simulink model "ARC_DTm"  (R2025b)
settings: Solver=FixedStepAuto  StartTime=0.0  StopTime=10080  FixedStep=1  RelTol=1e-3
PreLoadFcn:
  | %For Preload, set the working path
  | modelFolder = fileparts(which(bdroot));
  | addpath(genpath(modelFolder));
StartFcn:
  | tic
StopFcn:
  | fprintf("Sim Time: %.02f min", toc/60)
values from neighbouring files (symbols this model uses):
  batteryScenario = p.batteryScenario    [RUNSIM_ParameterSweep.m]    (also in _RUNSIM_ParameterSweep.m)
  Electricity_SalePriceModifier = 50/100    (= 0.5)    [RUNSIM_ParameterSweep.m]    (also in _RUNSIM_ParameterSweep.m)
  LUT = LUT_load.gamLUT    [RUNSIM_ParameterSweep.m]    (also in _RUNSIM_ParameterSweep.m)
  minimum_UF_system_flow = 5833    [RUNSIM_ParameterSweep.m]    (also in _RUNSIM_ParameterSweep.m)
  PROS1_recoveryrate = 61    [RUNSIM_ParameterSweep.m]    (also in _RUNSIM_ParameterSweep.m)
  PROS2_recoveryrate = 62    [RUNSIM_ParameterSweep.m]    (also in _RUNSIM_ParameterSweep.m)
  ROstabilization_time = p.ROstabilization_time    [RUNSIM_ParameterSweep.m]    (also in _RUNSIM_ParameterSweep.m)
  solarModifier = maximum_solar_generation / 300    [RUNSIM_ParameterSweep.m]    (also in _RUNSIM_ParameterSweep.m)
  TSRO_recoveryrate = 51    [RUNSIM_ParameterSweep.m]    (also in _RUNSIM_ParameterSweep.m)
  UF_RecoveryRate = 96    [RUNSIM_ParameterSweep.m]    (also in _RUNSIM_ParameterSweep.m)
undefined symbols (not defined in the file or in its folder): A_PROS1, A_PROS2, A_TSRO, B_PROS1, B_PROS2, B_TSRO, BW_Max_Time, BW_Max_Vol_gal, CEB_Max_Time, CEB_Max_Vol_gal, CIP_Max_Time, E, FF, h, L, w
libraries: simulink x40
(part 10 of 11)

== matlab function ARC_DTm/PROS2_4_Pump/MATLAB Function1 ==
  data: Q_des input; speed output; h_des input; power output
function [speed, power] = query_pump(Q_des, h_des)
% QUERY_PUMP Find pump speed, power, and efficiency given flow and head
%MUST UPDATE the pump_data call
%
% Inputs:
%   Q_des     - Desired flow rate (gpm)
%   h_des     - Desired added head (ft)
%   pump_data - Struct for a single pump (e.g. pump.pump_A)
%
% Outputs:
%   speed      - Interpolated speed
%   power      - Interpolated power
%   total_eff  - Interpolated total efficiency (%)
%   totalPower - Power demand accounting for efficiency (power / total_eff / 100)

persistent pump_data Q_min h_min speed_min  P_min
if isempty(pump_data)
    loaded = coder.load('Pumps\LookupTables.mat');
    pump_data = loaded.pump.RO_IS_pump;
    Q_min = min(pump_data.Q_grid(:));
    h_min = min(pump_data.H_grid(:));

    speed_min = interp2(pump_data.Q_grid, pump_data.H_grid, pump_data.speed_grid, Q_min, h_min, 'linear');
    P_min = interp2(pump_data.H_grid_pwr, pump_data.S_grid_pwr, pump_data.power_grid, h_min, speed_min, 'linear');

end

%zero flow conditions not present in the existing dataset.
if Q_des <= .1 * Q_min
    speed = 0;
    power = 0;
    total_eff = 0;
    return
end

% Normal lookup
speed = interp2(pump_data.Q_grid, pump_data.H_grid, ...
    pump_data.speed_grid, Q_des, h_des, 'linear');

if ~isnan(speed)
    power = interp2(pump_data.H_grid_pwr, pump_data.S_grid_pwr, ...
        pump_data.power_grid, h_des, speed, 'linear');
else
    power = NaN;
end

% Fallback only for low-end conditions
if isnan(speed) || isnan(power)
    if Q_des < Q_min       
        speed = speed_min / Q_min * Q_des;
         power = (speed / speed_min)^3 * P_min;

    else if h_des < h_min
        speed = speed_min * (h_des / h_min)^(1/2);
        power = (speed / speed_min)^3 * P_min;

    else
        speed = 0;
        power = 0;
    end


end


end

== matlab function ARC_DTm/PROS2_4/MATLAB Function1 ==
  data: W input; h input; dh output
function dh = hydDiameter(W,h)

dh = 2*h*W/(h+W);

== matlab function ARC_DTm/PROS2_4/MATLAB Function2 ==
  data: cperm input; cbrine output; Qperm input; Qbrine input; Qfeed input; cfeed input
function cbrine = fcn(cperm, Qperm, Qbrine, Qfeed, cfeed)

Wtot = Qfeed * cfeed;
Wperm = cperm * Qperm;

%account for NaN
if Qbrine > 0
cbrine = (Wtot - Wperm)/Qbrine;
else
    cbrine = 0;
end

== matlab function ARC_DTm/TSRO_Pump_1/MATLAB Function1 ==
  data: Q_des input; h_des input; power output
function power  = query_pump(Q_des, h_des)
% QUERY_PUMP Find pump speed, power, and efficiency given flow and head
%MUST UPDATE the pump_data call
%
% Inputs:
%   Q_des     - Desired flow rate (gpm)
%   h_des     - Desired added head (ft)
%   pump_data - Struct for a single pump (e.g. pump.pump_A)
%
% Outputs:
%   power      - Interpolated power
%   total_eff  - Interpolated total efficiency (%)
%   totalPower - Power demand accounting for efficiency (power / total_eff / 100)

persistent pump_data Q_min h_min P_min
if isempty(pump_data)
    loaded = coder.load('Pumps\LookupTables.mat');
    pump_data = loaded.pump.tsro;
    Q_min = min(pump_data.Q_grid(:));
    h_min = min(pump_data.H_grid(:));

    P_min = interp2(pump_data.Q_grid, pump_data.H_grid, pump_data.power_grid, h_min, Q_min, 'linear');

end

%zero flow conditions not present in the existing dataset.
if Q_des <= .1 * Q_min
    power = 0;
    return
end

% Normal lookup
power = interp2(pump_data.Q_grid, pump_data.H_grid, ...
    pump_data.power_grid, Q_des, h_des, 'linear');

if isnan(power)
    power = 0;
    return

end

== matlab function ARC_DTm/PROS2_4/Subsystem/MATLAB Function ==
  data: T input; Pfeed input; Pperm input; A input; B input; cfeed input; cperm_prev input; Jw_prev input; dh input; L input; u input; Jw output; cperm output; deltaPi_bar output
function [Jw, cperm, deltaPi_bar] = ROBehavior(T, Pfeed, Pperm, A, B, cfeed, cperm_prev,Jw_prev, dh, L, u)
   
    cmem = ConP(cfeed, T, dh, L, u, Jw_prev);
    [pi_feed] = osmPres(T,cmem);
    [pi_perm] = osmPres(T,cperm_prev);
    
    deltaPi_bar = pi_feed - pi_perm;
    [Jw, cperm] = solutionDiffusion(T, Pfeed, Pperm, A, B, cmem, cperm_prev, pi_feed, pi_perm);
end

== matlab function ARC_DTm/TSRO_1/MATLAB Function1 ==
  data: W input; h input; dh output
function dh = hydDiameter(W,h)

dh = 2*h*W/(h+W);

== matlab function ARC_DTm/TSRO_1/MATLAB Function2 ==
  data: cperm input; cbrine output; Qperm input; Qbrine input; Qfeed input; cfeed input
function cbrine = fcn(cperm, Qperm, Qbrine, Qfeed, cfeed)

Wtot = Qfeed * cfeed;
Wperm = cperm * Qperm;

%account for NaN
if Qbrine > 0
cbrine = (Wtot - Wperm)/Qbrine;
else
    cbrine = 0;
end

== matlab function ARC_DTm/TSRO_1/Subsystem/MATLAB Function ==
  data: T input; Pfeed input; Pperm input; A input; B input; cfeed input; cperm_prev input; Jw_prev input; dh input; L input; u input; Jw output; cperm output; deltaPi_bar output
function [Jw, cperm, deltaPi_bar] = ROBehavior(T, Pfeed, Pperm, A, B, cfeed, cperm_prev,Jw_prev, dh, L, u)
    
    
    cmem = ConP(cfeed, T, dh, L, u, Jw_prev);
    [pi_feed] = osmPres(T,cmem);
    [pi_perm] = osmPres(T,cperm_prev);
    deltaPi_bar = pi_feed - pi_perm;
    
    [Jw, cperm] = solutionDiffusion(T, Pfeed, Pperm, A, B, cmem, cperm_prev, pi_feed, pi_perm);
end

== matlab function ARC_DTm/TSRO_3/MATLAB Function1 ==
  data: W input; h input; dh output
function dh = hydDiameter(W,h)

dh = 2*h*W/(h+W);

== matlab function ARC_DTm/TSRO_3/MATLAB Function2 ==
  data: cperm input; cbrine output; Qperm input; Qbrine input; Qfeed input; cfeed input
function cbrine = fcn(cperm, Qperm, Qbrine, Qfeed, cfeed)

Wtot = Qfeed * cfeed;
Wperm = cperm * Qperm;

%account for NaN
if Qbrine > 0
cbrine = (Wtot - Wperm)/Qbrine;
else
    cbrine = 0;
end

== matlab function ARC_DTm/TSRO_3/Subsystem/MATLAB Function ==
  data: T input; Pfeed input; Pperm input; A input; B input; cfeed input; cperm_prev input; Jw_prev input; dh input; L input; u input; Jw output; cperm output; deltaPi_bar output
function [Jw, cperm, deltaPi_bar] = ROBehavior(T, Pfeed, Pperm, A, B, cfeed, cperm_prev,Jw_prev, dh, L, u)
    
    
    cmem = ConP(cfeed, T, dh, L, u, Jw_prev);

    [pi_feed] = osmPres(T,cmem);
    [pi_perm] = osmPres(T,cperm_prev);
    
    deltaPi_bar = pi_feed - pi_perm;
    [Jw, cperm] = solutionDiffusion(T, Pfeed, Pperm, A, B, cmem, cperm_prev, pi_feed, pi_perm);
end

== matlab function ARC_DTm/Product Water Tank/MATLAB Function ==
  settings: updateMethod=DISCRETE
  data: inflows input; newInflows output; outflows input; vol input; volStored input; upperVol input; lowerVol input; newOutflows output; dVdt output; t output; t input
function [newInflows, newOutflows, dVdt, t] = tankControllerLogic(inflows, outflows, vol, volStored, upperVol, lowerVol,t)
%determine tanks flows
inflowSum = sum(inflows); %total volume to be pushed into tank [FLOW]
outflowSum = sum(outflows); %total volume to be pulled from tank [FLOW]

%set timer to exist each time step
% persistent t
if isempty(t)
    t = 0;
end

if volStored >= upperVol
    t = 15;
elseif volStored <= lowerVol
    t = -15;
end


% disp("t = " + t)
%set flows to reach desired operating conditions
if t > 0 %reduce inflows
    newOutflows = outflows; %maintain outflows
    newInflows = zeros(length(inflows),1);
    inflowRatio = zeros(length(inflows),1); %preallocate variable
    newInflowSum = outflowSum * .95; %reduce Inflows to 95% outflows

    %maintain inflow ratios at new inflow level
    for i = 1:length(inflows)
        
        inflowRatio(i) = inflows(i)/inflowSum;
        newInflows(i) = newInflowSum * inflowRatio(i);
    end
    dVdt = newInflowSum - outflowSum;
    t = t-1; %reduce timer one step

elseif t < 0 %reduce outflows
    
    newInflows = inflows; %maintain inflows
  
    outflowRatio = zeros(length(outflows),1); %prellocate variable
    newOutflows = zeros(length(outflows),1);%preallocate variable
    newOutflowSum = inflowSum * .95; %reduce outflows to be below inflows

    %maintain inflow ratios at new inflow level
    for i = 1:length(outflows)
        outflowRatio(i) = outflows(i)/outflowSum;
        newOutflows(i) = newOutflowSum * outflowRatio(i);

    end
    dVdt = inflowSum - newOutflowSum;
    t = t+1; %reduce timer one step
    
else
    newInflows = inflows;
    newOutflows = outflows;
    dVdt = inflowSum - outflowSum;
end

%update stored volume

volStored = volStored + dVdt;

%if outside oeprating conditions, begin to adjust flows


end

== matlab function ARC_DTm/TSRO_2/MATLAB Function1 ==
  data: W input; h input; dh output
function dh = hydDiameter(W,h)

dh = 2*h*W/(h+W);

== matlab function ARC_DTm/TSRO_2/MATLAB Function2 ==
  data: cperm input; cbrine output; Qperm input; Qbrine input; Qfeed input; cfeed input
function cbrine = fcn(cperm, Qperm, Qbrine, Qfeed, cfeed)

Wtot = Qfeed * cfeed;
Wperm = cperm * Qperm;

%account for NaN
if Qbrine > 0
cbrine = (Wtot - Wperm)/Qbrine;
else
    cbrine = 0;
end

== matlab function ARC_DTm/TSRO_2/Subsystem/MATLAB Function ==
  data: T input; Pfeed input; Pperm input; A input; B input; cfeed input; cperm_prev input; Jw_prev input; dh input; L input; u input; Jw output; cperm output; deltaPi_bar output
function [Jw, cperm, deltaPi_bar] = ROBehavior(T, Pfeed, Pperm, A, B, cfeed, cperm_prev,Jw_prev, dh, L, u)
    
    
    cmem = ConP(cfeed, T, dh, L, u, Jw_prev);

    [pi_feed] = osmPres(T,cmem);
    [pi_perm] = osmPres(T,cperm_prev);
    
    deltaPi_bar = pi_feed - pi_perm;
    [Jw, cperm] = solutionDiffusion(T, Pfeed, Pperm, A, B, cmem, cperm_prev, pi_feed, pi_perm);
end

== matlab function ARC_DTm/TSRO_4/MATLAB Function1 ==
  data: W input; h input; dh output
function dh = hydDiameter(W,h)

dh = 2*h*W/(h+W);

== matlab function ARC_DTm/TSRO_4/MATLAB Function2 ==
  data: cperm input; cbrine output; Qperm input; Qbrine input; Qfeed input; cfeed input
function cbrine = fcn(cperm, Qperm, Qbrine, Qfeed, cfeed)

Wtot = Qfeed * cfeed;
Wperm = cperm * Qperm;

%account for NaN
if Qbrine > 0
cbrine = (Wtot - Wperm)/Qbrine;
else
    cbrine = 0;
end

== matlab function ARC_DTm/TSRO_4/Subsystem/MATLAB Function ==
  data: T input; Pfeed input; Pperm input; A input; B input; cfeed input; cperm_prev input; Jw_prev input; dh input; L input; u input; Jw output; cperm output; deltaPi_bar output
function [Jw, cperm, deltaPi_bar] = ROBehavior(T, Pfeed, Pperm, A, B, cfeed, cperm_prev,Jw_prev, dh, L, u)
    
    
    cmem = ConP(cfeed, T, dh, L, u, Jw_prev);

    [pi_feed] = osmPres(T,cmem);
    [pi_perm] = osmPres(T,cperm_prev);
    
    deltaPi_bar = pi_feed - pi_perm;
    [Jw, cperm] = solutionDiffusion(T, Pfeed, Pperm, A, B, cmem, cperm_prev, pi_feed, pi_perm);
end

== matlab function ARC_DTm/TSRO_Pump_3/MATLAB Function1 ==
  data: Q_des input; h_des input; power output
function power  = query_pump(Q_des, h_des)
% QUERY_PUMP Find pump speed, power, and efficiency given flow and head
%MUST UPDATE the pump_data call
%
% Inputs:
%   Q_des     - Desired flow rate (gpm)
%   h_des     - Desired added head (ft)
%   pump_data - Struct for a single pump (e.g. pump.pump_A)
%
% Outputs:
%   power      - Interpolated power
%   total_eff  - Interpolated total efficiency (%)
%   totalPower - Power demand accounting for efficiency (power / total_eff / 100)

persistent pump_data Q_min h_min P_min
if isempty(pump_data)
    loaded = coder.load('Pumps\LookupTables.mat');
    pump_data = loaded.pump.tsro;
    Q_min = min(pump_data.Q_grid(:));
    h_min = min(pump_data.H_grid(:));

    P_min = interp2(pump_data.Q_grid, pump_data.H_grid, pump_data.power_grid, h_min, Q_min, 'linear');

end

%zero flow conditions not present in the existing dataset.
if Q_des <= .1 * Q_min
    power = 0;
    return
end

% Normal lookup
power = interp2(pump_data.Q_grid, pump_data.H_grid, ...
    pump_data.power_grid, Q_des, h_des, 'linear');

if isnan(power)
    power = 0;
    return

end

== matlab function ARC_DTm/TSRO_Pump_4/MATLAB Function1 ==
  data: Q_des input; h_des input; power output
function power  = query_pump(Q_des, h_des)
% QUERY_PUMP Find pump speed, power, and efficiency given flow and head
%MUST UPDATE the pump_data call
%
% Inputs:
%   Q_des     - Desired flow rate (gpm)
%   h_des     - Desired added head (ft)
%   pump_data - Struct for a single pump (e.g. pump.pump_A)
%
% Outputs:
%   power      - Interpolated power
%   total_eff  - Interpolated total efficiency (%)
%   totalPower - Power demand accounting for efficiency (power / total_eff / 100)

persistent pump_data Q_min h_min P_min
if isempty(pump_data)
    loaded = coder.load('Pumps\LookupTables.mat');
    pump_data = loaded.pump.tsro;
    Q_min = min(pump_data.Q_grid(:));
    h_min = min(pump_data.H_grid(:));

    P_min = interp2(pump_data.Q_grid, pump_data.H_grid, pump_data.power_grid, h_min, Q_min, 'linear');

end

%zero flow conditions not present in the existing dataset.
if Q_des <= .1 * Q_min
    power = 0;
    return
end

% Normal lookup
power = interp2(pump_data.Q_grid, pump_data.H_grid, ...
    pump_data.power_grid, Q_des, h_des, 'linear');

if isnan(power)
    power = 0;
    return

end

== stateflow chart ARC_DTm/UF Maintenance Coordinator/Sample_Stateflows ==
  settings: sampleTime=1  executeAtInitialization=1
  note: Unit State Machine — FIFO Maintenance Dispatch
      | This chart controls a single filtration unit through four operational states: Standby, Running, Await_Maintenance, BW_Maintenance, and CEB_Maintenance.
      | The unit begins in Standby, awaiting a startup command from the central dispatcher. Once commanded on, it enters Running, where it operates normally and tracks cumulative downtime. If a maintenance request is triggered, the unit transitions to Await_Maintenance, remaining online until the dispatcher confirms it can be released.
      | Two maintenance sequences are supported. A Backwash (BW) is a fixed-duration event (4 timesteps). A Chemically Enhanced Backwash (CEB) is a stochastic event lasting between 30 and 90 timesteps, sampled from a uniform distribution at entry. CEB is always followed by a BW cycle.
      | Upon completion of maintenance, the unit returns to Standby and re-enters the startup queue at the back, consistent with FIFO dispatching logic.
  note: Unit_cmd = 1 for running, 0 for off.
  state Standby
    during:
    %Unit is off, but awaiting startup.
    unit_in_startup_queue = 1;
    unit_in_operation = 0;
    %Ensure that the maintenance resets are occuring.
    maintenance_completion_indicator = 0;
  state Running
    entry:
    %Reset downtime timer
    cycle_downtime = 0;
    during:
    %Unit on, not in maint queue.
    unit_in_operation = 1;
    unit_in_maint_queue = 0;
  state Await_standby
    %Unit , Enter maint Queue
    during:
    unit_in_operation = 0;
    unit_in_maint_queue = 1;
  state Await_maintenance
    %Unit stays on, Enter maint Queue
    during:
    unit_in_operation = 1;
    unit_in_maint_queue = 1;
  state CEB_Maintenance
    %Unit is in chemically enhanced backwash. After CEB, do BW.
    %At start, determine a maintenance time within a uniform range of 30-60 min.
    entry:
    needed_maint_time = 30 + (60-30) * rand();
    %Exit state when time in maintenance is >= expected time.
    during:
    unit_in_operation = -1; %unit in maintenance
    %update maintenance time every step.
    cycle_downtime = cycle_downtime + 1;
  state BW_Maintenance
    entry:
    needed_maint_time = 1.5;
    %Exit state when time in maintenance is >= expected time.
    during:
    unit_in_operation = -1; %unit in maintenance
    %update maintenance time every step.
    cycle_downtime = cycle_downtime + 1;
    %ensure that the CEB is not continually reseting.
    maintenance_completion_indicator = 0;
  note: Maintenance Completion Indicator represents a signal to reset the counters at the UF unit tracking backwash cycles (signal = 2) and time in operations (signal = 1). These are pulse signals that reset integrators.
  (default) -> Running
  Standby -> Running : [startup_cmd == 1]{unit_in_startup_queue = 0;}
  Running -> (junction 44) [order 2] : [standby_cmd == 1]
  Running -> Await_maintenance [order 1] : [maint_req ~=0]
  (junction 22) -> Standby
  Await_standby -> (junction 47) : [standby_cmd == 1 && maint_cmd == 1]
  (junction 47) -> (junction 11)
  (junction 44) -> Await_standby
  Await_maintenance -> (junction 11) [order 2] : [maint_req == 1 && maint_cmd == 1] {unit_in_maint_queue = 0;}
  (junction 11) -> BW_Maintenance
  Await_maintenance -> CEB_Maintenance [order 1] : [maint_req == 2 && maint_cmd ==1]
  CEB_Maintenance -> BW_Maintenance : [after(needed_maint_time, tick)]{maintenance_completion_indicator = 2;}
  BW_Maintenance -> (junction 22) : [after(needed_maint_time, tick)]
      | {maintenance_completion_indicator = 1;}
  data: maint_cmd input; maint_req input; standby_cmd input; startup_cmd input; unit_in_maint_queue output; unit_in_startup_queue output; cycle_downtime local; needed_maint_time local; unit_in_operation output; maintenance_completion_indicator output

== matlab function ARC_DTm/UF_Feed_Manifold/UF_Dispatcher ==
  data: flows output; max_flow_per_unit input; flow_actual input; Number_in_service output; flow_setpoint input; prev_flows input; demanded_flows output
function [flows, Number_in_service, demanded_flows] = UF_Dispatcher(max_flow_per_unit, flow_actual, flow_setpoint, prev_flows)

num_units_available = 10; 
flows = zeros( num_units_available,1);
demanded_flows = zeros(num_units_available,1);

current_units = sum(prev_flows>0);
target_units = min(ceil(flow_setpoint / max_flow_per_unit), num_units_available);
% Unit count driven by setpoint

    %during rampdown, avoid shutting off all units immediately
    if flow_setpoint == 0 && flow_actual ~= 0
        Number_in_service = max(target_units, current_units);
    else
        Number_in_service = target_units;
    end

% Target each unit is heading toward (based on setpoint)
demanded_flows(1:Number_in_service) = flow_setpoint / Number_in_service;

% Change in total actual flow this timestep (this should be throttled by
% rate limiter) on flow_actual.
delta_Q_total = flow_actual - sum(prev_flows); %total change in flow this timestep
avg_delta_Q_unit = delta_Q_total/Number_in_service; %benchmark to limit rate change.

% Distribute that delta evenly across active units, move toward demanded
delta_Q_unit_demanded = zeros(num_units_available,1); %demanded change in flows to reach setpoint
delta_Q = zeros(num_units_available,1); %actual change in flows this step.
for i = 1:num_units_available

        %get demanded change in flows.
        delta_Q_unit_demanded(i) = demanded_flows(i) - prev_flows(i);  
         
        delta_Q(i) = sign(delta_Q_unit_demanded(i)) * min(abs(delta_Q_unit_demanded(i)), abs(delta_Q_total/Number_in_service));


        flows(i) = prev_flows(i) + delta_Q(i);
        

        delta_Q_total = delta_Q_total - delta_Q(i);
end

end

== matlab function ARC_DTm/Product Water Tank/Tank Storage/Manage Overflows/Reduce to Zero ==
  data: u input; y output
function y = fcn(u)
    if u > 0 
        y = u -1;
        
    elseif u < 0
        y = u+1;
    else
        y = 0;
    end
    fprintf("Timer = ", +y)
end

== matlab function ARC_DTm/UF Maintenance Coordinator/UF_FIFO_Coordinator ==
  data: startup_req input size=[10 1]; maint_req input size=[10 1]; operating_states input; startup_cmd output size=[10 1]; flows input; maint_cmd output size=[10 1]; shutdown_cmd output size=[10 1]; assigned_flows output
function [startup_cmd, maint_cmd, shutdown_cmd,  assigned_flows] = ...
        FIFO_coordinator(startup_req, maint_req, operating_states, flows)
% ========================================
%  FIFO_coordinator  —  Startup / Maintenance / Shutdown coordinator
%
%  Manages 10 units so that exactly `demanded_units` are running at all
%  times. All queues are strict FIFO. Designed for use as a MATLAB
%  Function block inside Simulink (fixed-step discrete, Ts = 1).
%
%  INPUTS
%  startup_req   [10×1]  bool   unit is in Standby, requesting startup
%  maint_req   [10×1]  int    0=none, 1=BW request, 2=CEB request
%  unit_in_operation  [10×1]  int    -1=in active maint, 0=standby, 1=running/await_maint
%  demanded_units   scalar  int    how many units should be online right now
%
%  OUTPUTS
%  startup_cmd    [10×1]  bool  tell unit to leave Standby to Running
%  maint_cmd  [10×1]  bool  tell unit to leave Await_Maintenance to BW/CEB
%  shutdown_cmd  [10×1]  bool tell unit to leave Running to Standby
%  running_count  scalar int   number of units currently online (operation == 1)
%
%  UNIT STATE ENCODING (unit_in_operation)
%   1:  Running OR Await_Maintenance  (online, contributing to flow)
%   0:  Standby                       (offline, may be in startup queue)
%  -1:  BW_Maintenance or CEB_Maint  (offline, maintenance in progress)
%
%  COORDINATOR DECISION ORDER (each timestep):
%   1. Enqueue   — register new startup/maint requests into FIFO queues
%   2. Shed Load — if running_count > demanded, release maint or shutdown
%   3. Maint     — if slot open and safe, release front of maint queue
%   4. Startup   — if running_count < demanded, pop from startup queue
% ==================================

N = 10;
demanded_units = sum(flows>0); %from flow logic, determine number of units needed
% ── Persistent state (survives across Simulink timesteps) ─────────────────
persistent startup_queue;   % ordered list of unit indices awaiting startup
persistent maint_queue;     % ordered list of unit indices awaiting maintenance

if isempty(startup_queue)
    startup_queue = [];
    maint_queue   = [];
end



% ── Initialise output vectors ─────────────────────────────────────────────
startup_cmd  = zeros(N, 1);
maint_cmd = zeros(N, 1);
shutdown_cmd = zeros(N, 1);

% ── Derived counts from unit feedback signals ─────────────────────────────
running_count = sum(operating_states == 1);   % online units
active_maint_count = sum(operating_states == -1);  % unit in BW or CEB
% =======================
% STEP 1 — Add to queues
%   Add newly requesting units to the back of their respective queues.
%   Guards prevent double-enqueuing.
% ================================
for i = 1:N

    % Startup queue: unit must be in Standby (op==0) and not already queued
    if startup_req(i) && ~ismember(i, startup_queue) && operating_states(i) == 0
        startup_queue(end+1) = i;
    end

    % Maint queue: unit must be online (operating state ==1) and not already queued
    if maint_req(i) ~= 0 && ~ismember(i, maint_queue) && operating_states(i) == 1
        maint_queue(end+1) = i; 
    end

end

% =========================================================================
% STEP 2 — SHED LOAD
%   If too many units are online, bring count down to demanded_units.
%
%   Priority 1: units already in Await_Maintenance (maint_queue front)
%               , then issue maint_cmd immediately; they go offline with 0 flow.
%               Only possible if no other unit is currently in active maint
%               (one-at-a-time constraint).
%               After issuing maint_cmd, continue immediately to re-evaluate
%               the while condition — do NOT fall into shutdown branch.
%
%   Priority 2: pure Running units → issue shutdown_cmd (lowest index first
%               among units not in maint_queue, to preserve FIFO integrity).
%               already_shutdown tracks victims within this timestep since
%               unit_in_operation won't update until next step.
% =========================================================================
already_shutdown = zeros(N, 1);   % prevents double-shutdown in same timestep
already_maint    = zeros(N, 1);   % tracks units sent to maint this timestep
                                  % (unit_in_operation won't update until next
                                  %  step, so we must exclude them manually)

%Case 1. turn down requires shut down of units                                  
while running_count > demanded_units

    % Priority 1: shed via maint queue if slot is open
    if ~isempty(maint_queue) && active_maint_count == 0
        victim                = maint_queue(1);
        maint_queue(1)        = [];
        maint_cmd(victim)     = 1;
        already_maint(victim) = 1;   % exclude from shutdown candidates
        running_count         = running_count - 1;
        active_maint_count    = active_maint_count + 1;
        continue;   % re-evaluate while condition; skip shutdown branch
    end

    % Priority 2: shutdown lowest-index running unit not in maint queue
    %   Exclude units already sent to maint this step (still show op==1)
    candidates = find(operating_states == 1         & ...
                      ~ismember((1:N)', maint_queue) & ...
                      ~already_shutdown  & ...
                      ~already_maint);
    if ~isempty(candidates)
        victim   = candidates(1);
        shutdown_cmd(victim) = 1;
        already_shutdown(victim)= 1;
        startup_queue(startup_queue == victim) = [];
        running_count = running_count - 1;
    else
        break;   % nothing left to shed this step
    end

end

% =======================================================
% STEP 3 — RELEASE MAINTENANCE
%   Conditions to release the front of the maint queue:
%     a) at least one unit is in the maint queue
%     b) no unit is currently in active maintenance (one-at-a-time)
%     c) there is a replacement unit on standby
% =========================================================
if ~isempty(maint_queue) && ...
   ~isempty(startup_queue) &&...
   active_maint_count == 0  

    next_maint_unit = maint_queue(1);
    maint_queue(1) = [];
    maint_cmd(next_maint_unit)  = 1;

    next_startup_unit = startup_queue(1);
    startup_queue(1) = [];
    startup_cmd(next_startup_unit) = 1;
    active_maint_count = active_maint_count + 1;

    % active_maint_count would increment next step via unit feedback
    % also, running_count remains unchanged as a new unit comes online.

end



% ============================================
% STEP 4 — START UNITS
%   If running_count is below demand, pop from the front of the startup
%   queue and issue startup_cmd. Repeat until balanced or queue exhausted.
% =========================================================
while running_count < demanded_units && ~isempty(startup_queue)

    next_startup_unit = startup_queue(1);
    startup_queue(1)        = [];
    startup_cmd(next_startup_unit)  = 1;
    running_count           = running_count + 1;
    % unit_in_operation will rise to 1 next step via unit Stateflow

end

% =========================================================================
% STEP 5 - Assign Flows
% Based on flows vector, distribute the flows per unit to the units that
% are on. 
%===============================================================
assigned_flows = zeros(N,1); %initialize object

online_units = find(operating_states==1); %array of indices for online units

if isempty(online_units)
    assigned_flows = zeros(N,1);
else

flows_available = flows(flows>0); %flows by unit by dispatcher

number_to_assign = min(length(online_units), length(flows_available)); %only assign the minimum

for i = 1:number_to_assign
    assigned_flows(online_units(i)) = flows_available(i);
end

end

end % function

== matlab function ARC_DTm/PRO Concentrate Manifold/Number TSRO Units ==
  data: flows output; max_flow_per_unit input; flow_actual input; Number_in_service output; flow_setpoint input; prev_flows input; Stabilization_Time input; ROstabilization_time input
function [flows, Number_in_service] = TSROUnits(max_flow_per_unit, flow_actual, flow_setpoint, prev_flows, Stabilization_Time,ROstabilization_time)

flows = zeros( 4,1);
demanded_flows = zeros(4,1);

current_units = sum(prev_flows>0);
target_units = min(ceil(flow_setpoint / max_flow_per_unit), 4);
% Unit count driven by setpoint
if Stabilization_Time >= ROstabilization_time

    %during rampdown, avoid shutting off all units immediately
    if flow_setpoint == 0 && flow_actual ~= 0
        Number_in_service = max(target_units, current_units);
    else
        Number_in_service = target_units;
    end
else
    Number_in_service = 2;
end

% Target each unit is heading toward (based on setpoint)
demanded_flows(1:Number_in_service) = flow_setpoint / Number_in_service;

% Change in total actual flow this timestep (this should be throttled by
% rate limiter) on flow_actual.
delta_Q_total = flow_actual - sum(prev_flows); %total change in flow this timestep
avg_delta_Q_unit = delta_Q_total/Number_in_service; %benchmark to limit rate change.

% Distribute that delta evenly across active units, move toward demanded
delta_Q_unit_demanded = zeros(4,1); %demanded change in flows to reach setpoint
delta_Q = zeros(4,1); %actual change in flows this step.
for i = 1:4

        %get demanded change in flows.
        delta_Q_unit_demanded(i) = demanded_flows(i) - prev_flows(i);  
         
        delta_Q(i) = sign(delta_Q_unit_demanded(i)) * min(abs(delta_Q_unit_demanded(i)), abs(delta_Q_total/Number_in_service));


        flows(i) = prev_flows(i) + delta_Q(i);
        

        delta_Q_total = delta_Q_total - delta_Q(i);
end

end

== matlab function ARC_DTm/UF Maintenance Coordinator/UF_State_Tracker ==
  data: in_startup_queue output; in_maint_queue output; startup_cmd input; operations_states output; maint_cmd input; shutdown_cmd input; maint_req input; maintenance_completion_indicators output
function [ in_startup_queue, in_maint_queue,operations_states, maintenance_completion_indicators] = ...
          UF_Operating_States(startup_cmd, maint_cmd, shutdown_cmd, maint_req)
% UF Maintenance Tracker
%This function is a more efficient way to operate N identical stateflow
%diagrams representing UF maintenance cycles. 

%Note that the ordering of the queue is handled within the Coordinator
%function, and the persistence of queueing order is also contained there.
% -------------------------------------------------------------------------

% ___ Inputs - From Coordinator___
%   startup_cmd  [10x1] logical, move units in queue Standby to Running
%   maint_cmd [10x1] logical, move units in queue Await_Maint to Maintenance
%   shutdown_cmd [10x1] logical, move units in queue Running/Await_Maint to Standby

% ___Inputs - from units___
% maintenance_requests [10x1] state-based triggers. move units from Running
% to Await_Maint
%   [0 (no maint request), 1 (Backwash request), 2 (Chemically-Enahnced BW
%   Req)]

% ___OUTPUTS - to coordinator___
%   operation_states [10x1] int: -1=active maint, 0=standby, 1=online
%   startup_queue  [10x1] logical
%   maint_queue [10x1] logical

%___Outputs - to units___
%   maintenance_completion_indicators  [10x1] int: 0=none, 1=BW complete, 2=CEB complete

% ___Internal Vectors___
%   needed_maint_time [10x1] double, stochastic constants for the duration
%   of a maintenance activity.
%   time_in_maintenance_p [10x1] double, maintenance duration

% -------------------------------------------------------------------------

N = 10;

% operations state constants. Use doubles for MATLAB Function block compatibility.
STANDBY = 0;
RUNNING = 1;
AWAIT_MAINTENANCE = 2;
BW_MAINTENANCE = -1;
CEB_MAINTENANCE = -2;



%Define and initialize persistent variables
%Note, in simulink, persistent variables cannot be used as function outputs, only internal state variables
persistent operations_states_p;
persistent time_in_maintenance_p;
persistent needed_maint_time_p;


if isempty(operations_states_p)

    % all units start in Standby
    operations_states_p = zeros(N,1); 
    time_in_maintenance_p = zeros(N,1); 
    needed_maint_time_p = zeros(N,1);
    


end

% Initialize outputs each tick. Note that the queues are stored in the
% UFCoordinator Function
maintenance_completion_indicators = zeros(N,1);
in_maint_queue = zeros(N,1);
in_startup_queue = zeros(N,1); 

%for each unit
for i = 1:N
    
    %determine the operating state
    switch operations_states_p(i)

        case STANDBY %state == 0

            % Stateflow Standby/during equivalent:
            %   unit is off, awaiting startup.
            
            %while unit is in standby:

            operations_states_p(i) = STANDBY; %not operating
            in_startup_queue(i) = 1; %in startup queue
            in_maint_queue(i) = 0; %no maintenance request

            if startup_cmd(i)
                operations_states_p(i) = RUNNING;
                in_startup_queue(i) = 0;
            end

        case RUNNING %state == 1
            % Stateflow Running/entry and during equivalent:
            % unit online, not in maintenance queue.

            operations_states_p(i) = RUNNING; %in operation

            %not in any queue
            in_startup_queue(i) = 0;
            in_maint_queue(i) = 0;
            
            %when shutdown command (during rampdown) issued by coordinator
            if shutdown_cmd(i)

                operations_states_p(i) = STANDBY; %no longer operating
                in_startup_queue(i) = 1; %enter startup queue

            %If  unit hits maintenance threshold(s)
            elseif maint_req(i) ~= 0

                %send out maintenance request. 
                operations_states_p(i) = AWAIT_MAINTENANCE;
                in_maint_queue(i) = 1;
            end

        case AWAIT_MAINTENANCE
            % Unit remains online while waiting for coordinator permission.
            operations_states_p(i) = AWAIT_MAINTENANCE;

            %Only in maintenance queue
            in_startup_queue(i) = 0;
            in_maint_queue(i) = 1;

            % If the shutdown command is issued (such as during rampdown)
            if shutdown_cmd(i)
                
                %enter standby and remove self from maintenance queue
                operations_states_p(i) = STANDBY;
                operations_states_p(i) = 0;
                in_startup_queue(i) = 1;
                in_maint_queue(i) = 0;
            
            %Otherwise, if the command to enter maintenance is issued:
            elseif maint_cmd(i)
                in_maint_queue(i) = 0; %remove self from maintenance queue
                time_in_maintenance_p(i) = 0; %initialize time in maintenance tracker
                
                %if unit requested CEB maintenance
                if maint_req(i) == 2
                    operations_states_p(i) = CEB_MAINTENANCE; 
                    % Stateflow entry action:
                    %   needed_maint_time = 30 + (60-30)*rand();
                    needed_maint_time_p(i) = 30 + 30*rand(); %set time to 30-60 mins

                    %Otherwise, if BW is requested (more common)
                else
                    operations_states_p(i) = BW_MAINTENANCE;
                    % Stateflow entry action:
                    %   needed_maint_time = 1.5;
                    needed_maint_time_p(i) = 1.5;  %set time to ~2 min. 
                end
            end

        case CEB_MAINTENANCE
            % Active CEB: unit offline, downtime accumulates.
            operations_states_p(i) = CEB_MAINTENANCE;
            in_startup_queue(i) = 0;
            in_maint_queue(i) = 0;
            time_in_maintenance_p(i) = time_in_maintenance_p(i) + 1;

            if time_in_maintenance_p(i) >= needed_maint_time_p(i)
                % CEB complete; original chart indicates CEB is followed by BW.
                maintenance_completion_indicators(i) = 2;
                operations_states_p(i) = BW_MAINTENANCE;

                time_in_maintenance_p(i) = 0;
                needed_maint_time_p(i) = 1.5;
            end

        case BW_MAINTENANCE
            % Active BW: unit offline, downtime accumulates.
            operations_states_p(i) = BW_MAINTENANCE;
            in_startup_queue(i) = 0;
            in_maint_queue(i) = 0;
            time_in_maintenance_p(i) = time_in_maintenance_p(i) + 1;

            if time_in_maintenance_p(i) >= needed_maint_time_p(i)
                % BW complete; return to Standby/startup queue.
                maintenance_completion_indicators(i) = 1;
                operations_states_p(i) = STANDBY;
                time_in_maintenance_p(i) = 0;
                needed_maint_time_p(i) = 0;
            end

        otherwise
            % Defensive recovery for invalid state values.
            operations_states_p(i) = STANDBY;
            time_in_maintenance_p(i) = 0;
            needed_maint_time_p(i) = 0;
            operations_states_p(i) = 0;
            in_startup_queue(i) = 1;
            in_maint_queue(i) = 0;
    end
end

% Refresh diagnostic outputs after state updates.
operations_states = sign(operations_states_p);


end

== matlab function ARC_DTm/UF Maintenance Coordinator/arhive/MATLAB Function ==
  data: startup_req input size=[10 1]; maint_req input size=[10 1]; unit_in_operation input; startup_cmd output size=[10 1]; demanded_units input; maint_cmd output size=[10 1]; shutdown_cmd output size=[10 1]; running_count output
function [startup_cmd, maint_cmd, shutdown_cmd, running_count] = ...
        FIFO_coordinator(startup_req, maint_req, unit_in_operation, demanded_units)
% =========================================================================
%  FIFO_coordinator  —  Startup / Maintenance / Shutdown coordinator
%
%  Manages 10 units so that exactly `demanded_units` are running at all
%  times. All queues are strict FIFO. Designed for use as a MATLAB
%  Function block inside Simulink (fixed-step discrete, Ts = 1).
%
%  INPUTS
%  startup_req        [10×1]  bool   unit is in Standby, requesting startup
%  maint_req          [10×1]  int    0=none, 1=BW request, 2=CEB request
%  unit_in_operation  [10×1]  int    -1=in active maint, 0=standby, 1=running/await_maint
%  demanded_units     scalar  int    how many units should be online right now
%
%  OUTPUTS
%  startup_cmd        [10×1]  bool   tell unit to leave Standby → Running
%  maint_cmd          [10×1]  bool   tell unit to leave Await_Maintenance → BW/CEB
%  shutdown_cmd       [10×1]  bool   tell unit to leave Running → Standby
%  running_count      scalar  int    number of units currently online (operation == 1)
%
%  UNIT STATE ENCODING (unit_in_operation)
%   1:  Running OR Await_Maintenance  (online, contributing to flow)
%   0:  Standby                       (offline, may be in startup queue)
%  -1:  BW_Maintenance or CEB_Maint  (offline, maintenance in progress)
%
%  COORDINATOR DECISION ORDER (each timestep):
%   1. Enqueue   — register new startup/maint requests into FIFO queues
%   2. Shed Load — if running_count > demanded, release maint or shutdown
%   3. Maint     — if slot open and safe, release front of maint queue
%   4. Startup   — if running_count < demanded, pop from startup queue
% =========================================================================

N = 10;
% ── Persistent state (survives across Simulink timesteps) ─────────────────
persistent startup_queue;   % ordered list of unit indices awaiting startup
persistent maint_queue;     % ordered list of unit indices awaiting maintenance

if isempty(startup_queue)
    startup_queue = [];
    maint_queue   = [];
end



% ── Initialise output vectors ─────────────────────────────────────────────
startup_cmd  = false(N, 1);
maint_cmd    = false(N, 1);
shutdown_cmd = false(N, 1);

% ── Derived counts from unit feedback signals ─────────────────────────────
running_count      = sum(unit_in_operation == 1);   % online units
active_maint_count = sum(unit_in_operation == -1);  % units in BW or CEB

% =========================================================================
% STEP 1 — ENQUEUE
%   Add newly requesting units to the back of their respective queues.
%   Guards prevent double-enqueuing.
% =========================================================================
for i = 1:N

    % Startup queue: unit must be in Standby (op==0) and not already queued
    if startup_req(i) && ~ismember(i, startup_queue) && unit_in_operation(i) == 0
        startup_queue(end+1) = i; %#ok<AGROW>
    end

    % Maint queue: unit must be online (op==1) and not already queued
    if maint_req(i) ~= 0 && ~ismember(i, maint_queue) && unit_in_operation(i) == 1
        maint_queue(end+1) = i; %#ok<AGROW>
    end

end

% =========================================================================
% STEP 2 — SHED LOAD
%   If too many units are online, bring count down to demanded_units.
%
%   Priority 1: units already in Await_Maintenance (maint_queue front)
%               → issue maint_cmd immediately; they go offline with 0 flow.
%               Only possible if no other unit is currently in active maint
%               (one-at-a-time constraint).
%               After issuing maint_cmd, continue immediately to re-evaluate
%               the while condition — do NOT fall into shutdown branch.
%
%   Priority 2: pure Running units → issue shutdown_cmd (lowest index first
%               among units not in maint_queue, to preserve FIFO integrity).
%               already_shutdown tracks victims within this timestep since
%               unit_in_operation won't update until next step.
% =========================================================================
already_shutdown = false(N, 1);   % prevents double-shutdown in same timestep
already_maint    = false(N, 1);   % tracks units sent to maint this timestep
                                  % (unit_in_operation won't update until next
                                  %  step, so we must exclude them manually)

while running_count > demanded_units

    % Priority 1: shed via maint queue if slot is open
    if ~isempty(maint_queue) && active_maint_count == 0
        victim                = maint_queue(1);
        maint_queue(1)        = [];
        maint_cmd(victim)     = true;
        already_maint(victim) = true;   % exclude from shutdown candidates
        running_count         = running_count - 1;
        active_maint_count    = active_maint_count + 1;
        continue;   % re-evaluate while condition; skip shutdown branch
    end

    % Priority 2: shutdown lowest-index running unit not in maint queue
    %   Exclude units already sent to maint this step (still show op==1)
    candidates = find(unit_in_operation == 1         & ...
                      ~ismember((1:N)', maint_queue) & ...
                      ~already_shutdown              & ...
                      ~already_maint);
    if ~isempty(candidates)
        victim                   = candidates(1);
        shutdown_cmd(victim)     = true;
        already_shutdown(victim) = true;
        startup_queue(startup_queue == victim) = [];
        running_count            = running_count - 1;
    else
        break;   % nothing left to shed this step
    end

end

% =========================================================================
% STEP 3 — RELEASE MAINTENANCE
%   Conditions to release the front of the maint queue:
%     a) at least one unit is in the maint queue
%     b) no unit is currently in active maintenance (one-at-a-time)
%     c) releasing won't drop running_count below demanded_units
%        (the unit goes offline during maint)
% =========================================================================
if ~isempty(maint_queue)         && ...
   active_maint_count == 0       && ...
   (running_count - 1) >= demanded_units

    next_unit = maint_queue(1);
    maint_queue(1)        = [];
    maint_cmd(next_unit)  = true;
    running_count         = running_count - 1;
    % active_maint_count would increment next step via unit feedback

end

% =========================================================================
% STEP 4 — START UNITS
%   If running_count is below demand, pop from the front of the startup
%   queue and issue startup_cmd. Repeat until balanced or queue exhausted.
% =========================================================================
while running_count < demanded_units && ~isempty(startup_queue)

    next_unit = startup_queue(1);
    startup_queue(1)        = [];
    startup_cmd(next_unit)  = true;
    running_count           = running_count + 1;
    % unit_in_operation will rise to 1 next step via unit Stateflow

end

end % function

== stateflow chart ARC_DTm/UF Maintenance Coordinator/arhive/UF_Operation State_1/UF1_Maintenance State ==
  settings: sampleTime=1  executeAtInitialization=1
  note: Unit State Machine — FIFO Maintenance Dispatch
      | This chart controls a single filtration unit through four operational states: Standby, Running, Await_Maintenance, BW_Maintenance, and CEB_Maintenance.
      | The unit begins in Standby, awaiting a startup command from the central dispatcher. Once commanded on, it enters Running, where it operates normally and tracks cumulative downtime. If a maintenance request is triggered, the unit transitions to Await_Maintenance, remaining online until the dispatcher confirms it can be released.
      | Two maintenance sequences are supported. A Backwash (BW) is a fixed-duration event (4 timesteps). A Chemically Enhanced Backwash (CEB) is a stochastic event lasting between 30 and 90 timesteps, sampled from a uniform distribution at entry. CEB is always followed by a BW cycle.
      | Upon completion of maintenance, the unit returns to Standby and re-enters the startup queue at the back, consistent with FIFO dispatching logic.
  note: Unit_cmd = 1 for running, 0 for off.
  state Standby
    during:
    %Unit is off, but awaiting startup.
    unit_in_startup_queue = 1;
    unit_in_operation = 0;
    %Ensure that the maintenance resets are occuring.
    maintenance_completion_indicator = 0;
  state Running
    entry:
    %Reset downtime timer
    cycle_downtime = 0;
    during:
    %Unit on, not in maint queue.
    unit_in_operation = 1;
    unit_in_maint_queue = 0;
  state Await_standby
    %Unit , Enter maint Queue
    during:
    unit_in_operation = 0;
    unit_in_maint_queue = 1;
  state Await_maintenance
    %Unit stays on, Enter maint Queue
    during:
    unit_in_operation = 1;
    unit_in_maint_queue = 1;
  state CEB_Maintenance
    %Unit is in chemically enhanced backwash. After CEB, do BW.
    %At start, determine a maintenance time within a uniform range of 30-60 min.
    entry:
    needed_maint_time = 30 + (60-30) * rand();
    %Exit state when time in maintenance is >= expected time.
    during:
    unit_in_operation = -1; %unit in maintenance
    %update maintenance time every step.
    cycle_downtime = cycle_downtime + 1;
  state BW_Maintenance
    entry:
    needed_maint_time = 1.5;
    %Exit state when time in maintenance is >= expected time.
    during:
    unit_in_operation = -1; %unit in maintenance
    %update maintenance time every step.
    cycle_downtime = cycle_downtime + 1;
    %ensure that the CEB is not continually reseting.
    maintenance_completion_indicator = 0;
  note: Maintenance Completion Indicator represents a signal to reset the counters at the UF unit tracking backwash cycles (signal = 2) and time in operations (signal = 1). These are pulse signals that reset integrators.
  (default) -> Running
  Standby -> Running : [startup_cmd == 1]{unit_in_startup_queue = 0;}
  Running -> (junction 44) [order 2] : [standby_cmd == 1]
  Running -> Await_maintenance [order 1] : [maint_req ~=0]
  (junction 22) -> Standby
  Await_standby -> (junction 47) : [standby_cmd == 1 && maint_cmd == 1]
  (junction 47) -> (junction 11)
  (junction 44) -> Await_standby
  Await_maintenance -> (junction 11) [order 2] : [maint_req == 1 && maint_cmd == 1] {unit_in_maint_queue = 0;}
  (junction 11) -> BW_Maintenance
  Await_maintenance -> CEB_Maintenance [order 1] : [maint_req == 2 && maint_cmd ==1]
  CEB_Maintenance -> BW_Maintenance : [after(needed_maint_time, tick)]{maintenance_completion_indicator = 2;}
  BW_Maintenance -> (junction 22) : [after(needed_maint_time, tick)]
      | {maintenance_completion_indicator = 1;}
  data: maint_cmd input; maint_req input; standby_cmd input; startup_cmd input; unit_in_maint_queue output; unit_in_startup_queue output; cycle_downtime local; needed_maint_time local; unit_in_operation output; maintenance_completion_indicator output
